simulink model "ev_tms_v4_2022"  (R2023a)
settings: Solver=VariableStepAuto  StartTime=0.0  StopTime=inf  RelTol=1e-3  AbsTol=1e-3
model workspace: external: MATLAB File /Users/rossschrader/Documents/GitHub/RL_EV_TMS/blower_control/power_comparison/ev_tms_v4_params.m (data not in the file)
undefined symbols (not defined in the file): ac_onoff, battery_C1_LUT, battery_capacity_LUT, battery_cell_cp, battery_cell_mass, battery_Em_LUT, battery_N_cells, battery_Qe_init, battery_R0_LUT, battery_R1_LUT, battery_SOC_LUT, battery_T_init, battery_temperature_LUT, bulb, cabin_duct_area, cabin_T_init, chiller_area_primary, chiller_N_baffles, chiller_N_tubes, chiller_tube_D, chiller_tube_L, chiller_wall_conductivity, chiller_wall_thickness, compressor_rpm_LUT, condenser_air_area_flow, condenser_air_area_primary, condenser_W, condenser_wall_conductivity, condenser_wall_thickness, coolant_channel_D, coolant_pipe_D, coolant_T_init, coolant_tank_area, coolant_tank_volume, coolant_valve_D_ratio_max, coolant_valve_D_ratio_min, coolant_valve_displacement, coolant_valve_S_max, evaporator_air_area_flow, evaporator_air_area_primary, evaporator_P_target, evaporator_W, evaporator_wall_conductivity, evaporator_wall_thickness, outlet, pump_speed_max, radiator_air_area_flow, radiator_air_area_primary, radiator_W, radiator_wall_conductivity, radiator_wall_thickness, refrigerant_alpha_init, refrigerant_pipe_D, T_env, T_setpoint
libraries: fl_lib x221, nesl_utility x79, SimscapeFluids_lib x25, LiBatteryElements_lib x16, sdl_lib x3, slpidlib x2, simulink x1, rllib x1, autolibshared x1, SignalEditorBlockLib x1
(part 7 of 7)

== system ev_tms_v4_2022/Environment/Parallel-Serial Mode Valve/Battery Coolant Tank Heat Transfer ==
  Convective Heat Transfer : fl_lib/Thermal/Thermal Elements/Convective Heat Transfer  thermal_type=foundation.enum.constant_variable.constant  area=3 * coolant_tank_area m^2  heat_tr_coeff=20 W/(m^2 * K)  min_heat_tr_coeff=1e-3 W/(K*m^2)  T_specify=off  T_priority=None  T=0 K  T_nominal_specify=off  T_nominal_unit=K  T_nominal_value=1  Q_specify=off  Q_priority=None  Q=0 W  Q_nominal_specify=off  Q_nominal_unit=W  Q_nominal_value=1
  Convective Heat Transfer1 : fl_lib/Thermal/Thermal Elements/Convective Heat Transfer  thermal_type=foundation.enum.constant_variable.constant  area=3 * coolant_tank_area m^2  heat_tr_coeff=20 W/(m^2 * K)  min_heat_tr_coeff=1e-3 W/(K*m^2)  T_specify=off  T_priority=None  T=0 K  T_nominal_specify=off  T_nominal_unit=K  T_nominal_value=1  Q_specify=off  Q_priority=None  Q=0 W  Q_nominal_specify=off  Q_nominal_unit=W  Q_nominal_value=1
  Environment Temperature : fl_lib/Thermal/Thermal Sources/Controlled Temperature Source
  Simulink-PS Converter : nesl_utility/Simulink-PS Converter  PhysicalDomain=network_engine_domain  SubClassName=ps_input  LeftPortType=input  RightPortType=output  PseudoPeriodic=off  Frequencies=[]  NoiseDistribution=none  NoiseParameters=[]  Unit=degC  AffineConversion=on  FilteringAndDerivatives=provide  SimscapeFilterOrder=1  InputFilterTimeConstant=0.001  UdotUserProvided=0
  Thermal Reference : fl_lib/Thermal/Thermal Elements/Thermal Reference
  A : PMIOPort  Side=Left
  B : PMIOPort  Port=2  Side=Left
  wires:
  [T_env] -> Simulink-PS Converter/1
  connections:
  Environment Temperature/LConn1 -- Convective Heat Transfer/RConn1 -- Convective Heat Transfer1/RConn1
  Thermal Reference/LConn1 -- Environment Temperature/RConn2
  Simulink-PS Converter/RConn1 -- Environment Temperature/RConn1
  B/RConn1 -- Convective Heat Transfer1/LConn1
  Convective Heat Transfer/LConn1 -- A/RConn1

== system ev_tms_v4_2022/Environment/Parallel-Serial Mode Valve/Motor Coolant Tank Heat Transfer ==
  Convective Heat Transfer : fl_lib/Thermal/Thermal Elements/Convective Heat Transfer  thermal_type=foundation.enum.constant_variable.constant  area=3 * coolant_tank_area m^2  heat_tr_coeff=20 W/(m^2 * K)  min_heat_tr_coeff=1e-3 W/(K*m^2)  T_specify=off  T_priority=None  T=0 K  T_nominal_specify=off  T_nominal_unit=K  T_nominal_value=1  Q_specify=off  Q_priority=None  Q=0 W  Q_nominal_specify=off  Q_nominal_unit=W  Q_nominal_value=1
  Convective Heat Transfer1 : fl_lib/Thermal/Thermal Elements/Convective Heat Transfer  thermal_type=foundation.enum.constant_variable.constant  area=3 * coolant_tank_area m^2  heat_tr_coeff=20 W/(m^2 * K)  min_heat_tr_coeff=1e-3 W/(K*m^2)  T_specify=off  T_priority=None  T=0 K  T_nominal_specify=off  T_nominal_unit=K  T_nominal_value=1  Q_specify=off  Q_priority=None  Q=0 W  Q_nominal_specify=off  Q_nominal_unit=W  Q_nominal_value=1
  Environment Temperature : fl_lib/Thermal/Thermal Sources/Controlled Temperature Source
  Simulink-PS Converter : nesl_utility/Simulink-PS Converter  PhysicalDomain=network_engine_domain  SubClassName=ps_input  LeftPortType=input  RightPortType=output  PseudoPeriodic=off  Frequencies=[]  NoiseDistribution=none  NoiseParameters=[]  Unit=degC  AffineConversion=on  FilteringAndDerivatives=provide  SimscapeFilterOrder=1  InputFilterTimeConstant=0.001  UdotUserProvided=0
  Thermal Reference : fl_lib/Thermal/Thermal Elements/Thermal Reference
  A : PMIOPort  Side=Right
  B : PMIOPort  Port=2  Side=Right
  wires:
  [T_env] -> Simulink-PS Converter/1
  connections:
  Simulink-PS Converter/RConn1 -- Environment Temperature/RConn1
  Thermal Reference/LConn1 -- Environment Temperature/RConn2
  Convective Heat Transfer/RConn1 -- Environment Temperature/LConn1 -- Convective Heat Transfer1/RConn1
  B/RConn1 -- Convective Heat Transfer1/LConn1
  A/RConn1 -- Convective Heat Transfer/LConn1

== system ev_tms_v4_2022/Environment/Radiator/Ram Pressure ==
  1/2 : fl_lib/Physical Signals/Functions/PS Gain  gain=0.5
  Controlled Pressure Source (MA) : fl_lib/Moist Air/Sources/Controlled Pressure Source (MA)  power_spec=foundation.enum.power_spec.isentropic  area_A=cabin_duct_area m^2  area_B=cabin_duct_area m^2
      settings: InternalSimscapePortConfiguration="{\"Bottom\":[],\"Left\":[{\"id\":\"A\",\"label\":\"A\",\"type\":\"foundation.moist_air.moist_air\"},{\"id\":\"P\",\"label\":\"P\",\"type\":\"input\"}],\"Right\":[{\"id\":\"B\",\"label\":\"B\",\"type\":\"foundation.moist_air.moist_air\"}],\"Top\":[]}"
  PS Product : fl_lib/Physical Signals/Functions/PS Product
  Thermodynamic Properties Sensor (MA) : fl_lib/Moist Air/Sensors/Thermodynamic Properties Sensor (MA)  measurement_mass_spec=foundation.enum.measurement_mass_spec.mixture  enthalpy=true  density=true  specific_heat=true  entropy=true
      settings: InternalSimscapePortConfiguration="{\"Bottom\":[{\"id\":\"CP\",\"label\":\"cp\",\"type\":\"output\"},{\"id\":\"S\",\"label\":\"s\",\"type\":\"output\"}],\"Left\":[{\"id\":\"A\",\"label\":\"A\",\"type\":\"foundation.moist_air.moist_air\"}],\"Right\":[{\"id\":\"H\",\"label\":\"h\",\"type\":\"output\"},{\"id\":\"RHO\",\"label\":\"ρ\",\"type\":\"output\"}],\"Top\":[]}"
  sqr : fl_lib/Physical Signals/Functions/PS Math Function  fcn_choice=foundation.enum.math_function.square  v=1
  A : PMIOPort  Side=Left
  V : PMIOPort  Port=2  Side=Left
  B : PMIOPort  Port=3  Side=Right
  connections:
  Controlled Pressure Source (MA)/RConn1 -- B/RConn1
  Controlled Pressure Source (MA)/LConn1 -- A/RConn1 -- Thermodynamic Properties Sensor (MA)/LConn1
  PS Product/RConn1 -- Controlled Pressure Source (MA)/LConn2
  1/2/RConn1 -- PS Product/LConn1
  sqr/RConn1 -- 1/2/LConn1
  V/RConn1 -- sqr/LConn1
  Thermodynamic Properties Sensor (MA)/RConn2 -- PS Product/LConn2

== system ev_tms_v4_2022/Environment/Radiator/SC1 ==
  Absolute Reference (TL) : fl_lib/Thermal Liquid/Elements/Absolute Reference (TL)
  Mass & Energy Flow Rate Sensor (TL) : fl_lib/Thermal Liquid/Sensors/Flow Rate Sensor (TL)  mass_flow_measure=true  volumetric_flow_measure=false  energy_flow_measure=true
      settings: InternalSimscapePortConfiguration="{\"Bottom\":[{\"id\":\"PHI\",\"label\":\"φ\",\"type\":\"output\"}],\"Left\":[{\"id\":\"A\",\"label\":\"A\",\"type\":\"foundation.thermal_liquid.thermal_liquid\"}],\"Right\":[{\"id\":\"B\",\"label\":\"B\",\"type\":\"foundation.thermal_liquid.thermal_liquid\"},{\"id\":\"M\",\"label\":\"M\",\"type\":\"output\"}],\"Top\":[]}"
  PS-Simulink Converter : nesl_utility/PS-Simulink Converter  PhysicalDomain=network_engine_domain  SubClassName=ps_output  LeftPortType=input  RightPortType=output  PseudoPeriodic=off  Frequencies=[]  VectorFormat=1-D array  Unit=W  AffineConversion=off
  Pressure & Temperature Sensor (TL) : fl_lib/Thermal Liquid/Sensors/Pressure & Temperature Sensor (TL)  reference=foundation.enum.MeasurementReference.difference  pressure=true  pressure_spec=foundation.enum.PressureMeasementSpec.Absolute  temperature=true
      settings: InternalSimscapePortConfiguration="{\"Bottom\":[{\"id\":\"T\",\"label\":\"T\",\"type\":\"output\"}],\"Left\":[{\"id\":\"A\",\"label\":\"A\",\"type\":\"foundation.thermal_liquid.thermal_liquid\"}],\"Right\":[{\"id\":\"B\",\"label\":\"B\",\"type\":\"foundation.thermal_liquid.thermal_liquid\"},{\"id\":\"P\",\"label\":\"P\",\"type\":\"output\"}],\"Top\":[]}"
  B : PMIOPort  Side=Left
  A : PMIOPort  Port=2  Side=Right
  tag scope: Phi_rad_in=global
  wires:
  PS-Simulink Converter/1 -> [Phi_rad_in]
  connections:
  Pressure & Temperature Sensor (TL)/LConn1 -- A/RConn1 -- Mass & Energy Flow Rate Sensor (TL)/LConn1
  Mass & Energy Flow Rate Sensor (TL)/RConn1 -- B/RConn1
  Absolute Reference (TL)/LConn1 -- Pressure & Temperature Sensor (TL)/RConn1
  Mass & Energy Flow Rate Sensor (TL)/RConn3 -- PS-Simulink Converter/LConn1

== system ev_tms_v4_2022/Environment/Radiator/SC2 ==
  Absolute Reference (TL) : fl_lib/Thermal Liquid/Elements/Absolute Reference (TL)
  Mass & Energy Flow Rate Sensor (TL) : fl_lib/Thermal Liquid/Sensors/Flow Rate Sensor (TL)  mass_flow_measure=true  volumetric_flow_measure=false  energy_flow_measure=true
      settings: InternalSimscapePortConfiguration="{\"Bottom\":[{\"id\":\"PHI\",\"label\":\"φ\",\"type\":\"output\"}],\"Left\":[{\"id\":\"A\",\"label\":\"A\",\"type\":\"foundation.thermal_liquid.thermal_liquid\"}],\"Right\":[{\"id\":\"B\",\"label\":\"B\",\"type\":\"foundation.thermal_liquid.thermal_liquid\"},{\"id\":\"M\",\"label\":\"M\",\"type\":\"output\"}],\"Top\":[]}"
  PS-Simulink Converter : nesl_utility/PS-Simulink Converter  PhysicalDomain=network_engine_domain  SubClassName=ps_output  LeftPortType=input  RightPortType=output  PseudoPeriodic=off  Frequencies=[]  VectorFormat=1-D array  Unit=W  AffineConversion=off
  Pressure & Temperature Sensor (TL) : fl_lib/Thermal Liquid/Sensors/Pressure & Temperature Sensor (TL)  reference=foundation.enum.MeasurementReference.difference  pressure=true  pressure_spec=foundation.enum.PressureMeasementSpec.Absolute  temperature=true
      settings: InternalSimscapePortConfiguration="{\"Bottom\":[{\"id\":\"T\",\"label\":\"T\",\"type\":\"output\"}],\"Left\":[{\"id\":\"A\",\"label\":\"A\",\"type\":\"foundation.thermal_liquid.thermal_liquid\"}],\"Right\":[{\"id\":\"B\",\"label\":\"B\",\"type\":\"foundation.thermal_liquid.thermal_liquid\"},{\"id\":\"P\",\"label\":\"P\",\"type\":\"output\"}],\"Top\":[]}"
  B : PMIOPort  Side=Left
  A : PMIOPort  Port=2  Side=Right
  tag scope: Phi_rad_out=global
  wires:
  PS-Simulink Converter/1 -> [Phi_rad_out]
  connections:
  Pressure & Temperature Sensor (TL)/LConn1 -- A/RConn1 -- Mass & Energy Flow Rate Sensor (TL)/LConn1
  Mass & Energy Flow Rate Sensor (TL)/RConn1 -- B/RConn1
  Absolute Reference (TL)/LConn1 -- Pressure & Temperature Sensor (TL)/RConn1
  Mass & Energy Flow Rate Sensor (TL)/RConn3 -- PS-Simulink Converter/LConn1

== system ev_tms_v4_2022/Reward/Temp Reward/If Action Subsystem11 ==
  Action Port : ActionPort  ActionPortLabel=else
  Constant : Constant  Value=15
  Out1 : Outport
  wires:
  Constant/1 -> Out1/1

== system ev_tms_v4_2022/Reward/Temp Reward/If Action Subsystem9 ==
  Input : Inport
  Action Port : ActionPort  ActionPortLabel=if(u1 > 0.5)
  Add : Sum
  Constant : Constant  Value=-10
  Gain : Gain  Gain=-10
  Out1 : Outport
  wires:
  Input/1 -> Gain/1
  Gain/1 -> Add/1
  Constant/1 -> Add/2
  Add/1 -> Out1/1

== system ev_tms_v4_2022/Scenario/Power Demand/Derivative ==
  V : Inport
  Gain : Gain  Gain=tau
  Integrator : Integrator
  Sum : Sum  Inputs=|+-
  A : Outport
  wires:
  V/1 -> Sum/1
  Sum/1 -> Gain/1
  Gain/1 -> Integrator/1, A/1
  Integrator/1 -> Sum/2

== system ev_tms_v4_2022/Controls/Fan Control/Condenser Requirement/Relay Level 1 ==
  in : Inport
  high : Inport  Port=2
  low : Inport  Port=3
  Data Type Conversion : DataTypeConversion  SaturateOnIntegerOverflow=off  RndMeth=Floor
  Relational Operator : RelationalOperator  OutDataTypeStr=boolean  RndMeth=Simplest  InputSameDT=off
  Relational Operator1 : RelationalOperator  Operator=>  OutDataTypeStr=boolean  RndMeth=Simplest  InputSameDT=off
  Relay : Relay  OnSwitchValue=1.5  OffSwitchValue=0.5
  Sum : Sum  Inputs=|++
  out : Outport
  wires:
  Sum/1 -> Data Type Conversion/1
  Data Type Conversion/1 -> Relay/1
  Relational Operator1/1 -> Sum/2
  Relational Operator/1 -> Sum/1
  Relay/1 -> out/1
  low/1 -> Relational Operator1/2
  high/1 -> Relational Operator/2
  in/1 -> Relational Operator/1, Relational Operator1/1

== system ev_tms_v4_2022/Controls/Fan Control/Condenser Requirement/Relay Level 2 ==
  in : Inport
  high : Inport  Port=2
  low : Inport  Port=3
  Data Type Conversion : DataTypeConversion  SaturateOnIntegerOverflow=off  RndMeth=Floor
  Relational Operator : RelationalOperator  OutDataTypeStr=boolean  RndMeth=Simplest  InputSameDT=off
  Relational Operator1 : RelationalOperator  Operator=>  OutDataTypeStr=boolean  RndMeth=Simplest  InputSameDT=off
  Relay : Relay  OnSwitchValue=1.5  OffSwitchValue=0.5
  Sum : Sum  Inputs=|++
  out : Outport
  wires:
  Sum/1 -> Data Type Conversion/1
  Data Type Conversion/1 -> Relay/1
  Relational Operator1/1 -> Sum/2
  Relational Operator/1 -> Sum/1
  Relay/1 -> out/1
  low/1 -> Relational Operator1/2
  high/1 -> Relational Operator/2
  in/1 -> Relational Operator/1, Relational Operator1/1

== system ev_tms_v4_2022/Controls/Fan Control/Condenser Requirement/Relay Level 3 ==
  in : Inport
  high : Inport  Port=2
  low : Inport  Port=3
  Data Type Conversion : DataTypeConversion  SaturateOnIntegerOverflow=off  RndMeth=Floor
  Relational Operator : RelationalOperator  OutDataTypeStr=boolean  RndMeth=Simplest  InputSameDT=off
  Relational Operator1 : RelationalOperator  Operator=>  OutDataTypeStr=boolean  RndMeth=Simplest  InputSameDT=off
  Relay : Relay  OnSwitchValue=1.5  OffSwitchValue=0.5
  Sum : Sum  Inputs=|++
  out : Outport
  wires:
  Sum/1 -> Data Type Conversion/1
  Data Type Conversion/1 -> Relay/1
  Relational Operator1/1 -> Sum/2
  Relational Operator/1 -> Sum/1
  Relay/1 -> out/1
  low/1 -> Relational Operator1/2
  high/1 -> Relational Operator/2
  in/1 -> Relational Operator/1, Relational Operator1/1

== system ev_tms_v4_2022/Environment/Battery/Pack 1/Lithium Cell 1RC ==
  note: Power
      | Losses
  C1 : LiBatteryElements_lib/C_table  C_Table=C1_LUT F  SOC_Table=SOC_LUT  Temp_Table=Temperature_LUT K  v0=0 V
      settings: InternalSimscapePortConfiguration="{\"Bottom\":[],\"Left\":[{\"id\":\"p\",\"label\":\"+\",\"type\":\"foundation.electrical.electrical\"},{\"id\":\"T\",\"label\":\"T\",\"type\":\"input\"},{\"id\":\"SOC\",\"label\":\"SOC\",\"type\":\"input\"}],\"Right\":[{\"id\":\"n\",\"label\":\"-\",\"type\":\"foundation.electrical.electrical\"}],\"Top\":[]}"
  Em_table : LiBatteryElements_lib/Em_table  C_Table=Capacity_LUT hr*A  Em_Table=Em_LUT V  SOC_Table=SOC_LUT  Temp_Table=Temperature_LUT K  Qinit=Qe_init hr*A
      settings: InternalSimscapePortConfiguration="{\"Bottom\":[],\"Left\":[{\"id\":\"p\",\"label\":\"+\",\"type\":\"foundation.electrical.electrical\"},{\"id\":\"C\",\"label\":\"C\",\"type\":\"output\"},{\"id\":\"SOC\",\"label\":\"SOC\",\"type\":\"output\"}],\"Right\":[{\"id\":\"n\",\"label\":\"-\",\"type\":\"foundation.electrical.electrical\"},{\"id\":\"T\",\"label\":\"T\",\"type\":\"input\"}],\"Top\":[]}"
  Power Sum : fl_lib/Physical Signals/Functions/PS Add
  R0 : LiBatteryElements_lib/R_table  R_Table=R0_LUT Ohm  SOC_Table=SOC_LUT  Temp_Table=Temperature_LUT K
      settings: InternalSimscapePortConfiguration="{\"Bottom\":[],\"Left\":[{\"id\":\"p\",\"label\":\"+\",\"type\":\"foundation.electrical.electrical\"},{\"id\":\"T\",\"label\":\"T\",\"type\":\"input\"},{\"id\":\"SOC\",\"label\":\"SOC\",\"type\":\"input\"}],\"Right\":[{\"id\":\"n\",\"label\":\"-\",\"type\":\"foundation.electrical.electrical\"},{\"id\":\"pow\",\"label\":\"POW\",\"type\":\"output\"}],\"Top\":[]}"
  R1 : LiBatteryElements_lib/R_table  R_Table=R1_LUT Ohm  SOC_Table=SOC_LUT  Temp_Table=Temperature_LUT K
      settings: InternalSimscapePortConfiguration="{\"Bottom\":[],\"Left\":[{\"id\":\"p\",\"label\":\"+\",\"type\":\"foundation.electrical.electrical\"},{\"id\":\"T\",\"label\":\"T\",\"type\":\"input\"},{\"id\":\"SOC\",\"label\":\"SOC\",\"type\":\"input\"}],\"Right\":[{\"id\":\"n\",\"label\":\"-\",\"type\":\"foundation.electrical.electrical\"},{\"id\":\"pow\",\"label\":\"POW\",\"type\":\"output\"}],\"Top\":[]}"
  P : PMIOPort  Side=Left
  + : PMIOPort  Port=2  Side=Left
  T : PMIOPort  Port=3  Side=Right
  - : PMIOPort  Port=4  Side=Right
  connections:
  R1/RConn2 -- Power Sum/LConn1
  Power Sum/LConn2 -- R0/RConn2
  P/RConn1 -- Power Sum/RConn1
  +/RConn1 -- R0/RConn1
  T/RConn1 -- Em_table/RConn2 -- R0/LConn2 -- C1/LConn2 -- R1/LConn2
  Em_table/LConn1 -- C1/LConn1 -- R1/LConn1
  C1/RConn1 -- R1/RConn1 -- R0/LConn1
  Em_table/RConn1 -- -/RConn1
  C1/LConn3 -- Em_table/LConn3 -- R1/LConn3 -- R0/LConn3

== system ev_tms_v4_2022/Environment/Battery/Pack 1/Thermal Model ==
  Battery Thermal Mass : fl_lib/Thermal/Thermal Elements/Thermal Mass  mass_type=foundation.enum.constant_variable.constant  mass=cell_mass*Ncells kg  sp_heat=cell_Cp_heat J/kg/K  mass_min=1e-6 kg  num_ports=foundation.enum.numPorts2.one  m_specify=off  m_priority=High  m=1 kg  m_nominal_specify=off  m_nominal_unit=kg  m_nominal_value=1  T_specify=on  T_priority=High  T=T_init K  T_nominal_specify=off  T_nominal_unit=K  T_nominal_value=1  Q_specify=off  Q_priority=None  Q=0 W  Q_nominal_specify=off  Q_nominal_unit=W  Q_nominal_value=1
  Controlled Heat Flow Rate Source : fl_lib/Thermal/Thermal Sources/Controlled Heat Flow Rate Source
  Temperature Sensor : fl_lib/Thermal/Thermal Sensors/Temperature Sensor  temperature_measure=foundation.enum.MeasurementReference.difference
  Thermal Reference : fl_lib/Thermal/Thermal Elements/Thermal Reference
  Thermal Reference2 : fl_lib/Thermal/Thermal Elements/Thermal Reference
  H : PMIOPort  Side=Left
  Pxn : PMIOPort  Port=2  Side=Left
  T : PMIOPort  Port=3  Side=Right
  connections:
  H/RConn1 -- Controlled Heat Flow Rate Source/LConn1 -- Battery Thermal Mass/LConn1 -- Temperature Sensor/LConn1
  Pxn/RConn1 -- Controlled Heat Flow Rate Source/RConn1
  Controlled Heat Flow Rate Source/RConn2 -- Thermal Reference2/LConn1
  Thermal Reference/LConn1 -- Temperature Sensor/RConn1
  T/RConn1 -- Temperature Sensor/RConn2

== system ev_tms_v4_2022/Environment/Battery/Pack 2/Lithium Cell 1RC ==
  note: Power
      | Losses
  C1 : LiBatteryElements_lib/C_table  C_Table=C1_LUT F  SOC_Table=SOC_LUT  Temp_Table=Temperature_LUT K  v0=0 V
      settings: InternalSimscapePortConfiguration="{\"Bottom\":[],\"Left\":[{\"id\":\"p\",\"label\":\"+\",\"type\":\"foundation.electrical.electrical\"},{\"id\":\"T\",\"label\":\"T\",\"type\":\"input\"},{\"id\":\"SOC\",\"label\":\"SOC\",\"type\":\"input\"}],\"Right\":[{\"id\":\"n\",\"label\":\"-\",\"type\":\"foundation.electrical.electrical\"}],\"Top\":[]}"
  Em_table : LiBatteryElements_lib/Em_table  C_Table=Capacity_LUT hr*A  Em_Table=Em_LUT V  SOC_Table=SOC_LUT  Temp_Table=Temperature_LUT K  Qinit=Qe_init hr*A
      settings: InternalSimscapePortConfiguration="{\"Bottom\":[],\"Left\":[{\"id\":\"p\",\"label\":\"+\",\"type\":\"foundation.electrical.electrical\"},{\"id\":\"C\",\"label\":\"C\",\"type\":\"output\"},{\"id\":\"SOC\",\"label\":\"SOC\",\"type\":\"output\"}],\"Right\":[{\"id\":\"n\",\"label\":\"-\",\"type\":\"foundation.electrical.electrical\"},{\"id\":\"T\",\"label\":\"T\",\"type\":\"input\"}],\"Top\":[]}"
  Power Sum : fl_lib/Physical Signals/Functions/PS Add
  R0 : LiBatteryElements_lib/R_table  R_Table=R0_LUT Ohm  SOC_Table=SOC_LUT  Temp_Table=Temperature_LUT K
      settings: InternalSimscapePortConfiguration="{\"Bottom\":[],\"Left\":[{\"id\":\"p\",\"label\":\"+\",\"type\":\"foundation.electrical.electrical\"},{\"id\":\"T\",\"label\":\"T\",\"type\":\"input\"},{\"id\":\"SOC\",\"label\":\"SOC\",\"type\":\"input\"}],\"Right\":[{\"id\":\"n\",\"label\":\"-\",\"type\":\"foundation.electrical.electrical\"},{\"id\":\"pow\",\"label\":\"POW\",\"type\":\"output\"}],\"Top\":[]}"
  R1 : LiBatteryElements_lib/R_table  R_Table=R1_LUT Ohm  SOC_Table=SOC_LUT  Temp_Table=Temperature_LUT K
      settings: InternalSimscapePortConfiguration="{\"Bottom\":[],\"Left\":[{\"id\":\"p\",\"label\":\"+\",\"type\":\"foundation.electrical.electrical\"},{\"id\":\"T\",\"label\":\"T\",\"type\":\"input\"},{\"id\":\"SOC\",\"label\":\"SOC\",\"type\":\"input\"}],\"Right\":[{\"id\":\"n\",\"label\":\"-\",\"type\":\"foundation.electrical.electrical\"},{\"id\":\"pow\",\"label\":\"POW\",\"type\":\"output\"}],\"Top\":[]}"
  P : PMIOPort  Side=Left
  + : PMIOPort  Port=2  Side=Left
  T : PMIOPort  Port=3  Side=Right
  - : PMIOPort  Port=4  Side=Right
  connections:
  R1/RConn2 -- Power Sum/LConn1
  Power Sum/LConn2 -- R0/RConn2
  P/RConn1 -- Power Sum/RConn1
  +/RConn1 -- R0/RConn1
  T/RConn1 -- Em_table/RConn2 -- R0/LConn2 -- C1/LConn2 -- R1/LConn2
  Em_table/LConn1 -- C1/LConn1 -- R1/LConn1
  C1/RConn1 -- R1/RConn1 -- R0/LConn1
  Em_table/RConn1 -- -/RConn1
  C1/LConn3 -- Em_table/LConn3 -- R1/LConn3 -- R0/LConn3

== system ev_tms_v4_2022/Environment/Battery/Pack 2/Thermal Model ==
  Battery Thermal Mass : fl_lib/Thermal/Thermal Elements/Thermal Mass  mass_type=foundation.enum.constant_variable.constant  mass=cell_mass*Ncells kg  sp_heat=cell_Cp_heat J/kg/K  mass_min=1e-6 kg  num_ports=foundation.enum.numPorts2.one  m_specify=off  m_priority=High  m=1 kg  m_nominal_specify=off  m_nominal_unit=kg  m_nominal_value=1  T_specify=on  T_priority=High  T=T_init K  T_nominal_specify=off  T_nominal_unit=K  T_nominal_value=1  Q_specify=off  Q_priority=None  Q=0 W  Q_nominal_specify=off  Q_nominal_unit=W  Q_nominal_value=1
  Controlled Heat Flow Rate Source : fl_lib/Thermal/Thermal Sources/Controlled Heat Flow Rate Source
  Temperature Sensor : fl_lib/Thermal/Thermal Sensors/Temperature Sensor  temperature_measure=foundation.enum.MeasurementReference.difference
  Thermal Reference : fl_lib/Thermal/Thermal Elements/Thermal Reference
  Thermal Reference2 : fl_lib/Thermal/Thermal Elements/Thermal Reference
  H : PMIOPort  Side=Left
  Pxn : PMIOPort  Port=2  Side=Left
  T : PMIOPort  Port=3  Side=Right
  connections:
  H/RConn1 -- Controlled Heat Flow Rate Source/LConn1 -- Battery Thermal Mass/LConn1 -- Temperature Sensor/LConn1
  Pxn/RConn1 -- Controlled Heat Flow Rate Source/RConn1
  Controlled Heat Flow Rate Source/RConn2 -- Thermal Reference2/LConn1
  Thermal Reference/LConn1 -- Temperature Sensor/RConn1
  T/RConn1 -- Temperature Sensor/RConn2

== system ev_tms_v4_2022/Environment/Battery/Pack 3/Lithium Cell 1RC ==
  note: Power
      | Losses
  C1 : LiBatteryElements_lib/C_table  C_Table=C1_LUT F  SOC_Table=SOC_LUT  Temp_Table=Temperature_LUT K  v0=0 V
      settings: InternalSimscapePortConfiguration="{\"Bottom\":[],\"Left\":[{\"id\":\"p\",\"label\":\"+\",\"type\":\"foundation.electrical.electrical\"},{\"id\":\"T\",\"label\":\"T\",\"type\":\"input\"},{\"id\":\"SOC\",\"label\":\"SOC\",\"type\":\"input\"}],\"Right\":[{\"id\":\"n\",\"label\":\"-\",\"type\":\"foundation.electrical.electrical\"}],\"Top\":[]}"
  Em_table : LiBatteryElements_lib/Em_table  C_Table=Capacity_LUT hr*A  Em_Table=Em_LUT V  SOC_Table=SOC_LUT  Temp_Table=Temperature_LUT K  Qinit=Qe_init hr*A
      settings: InternalSimscapePortConfiguration="{\"Bottom\":[],\"Left\":[{\"id\":\"p\",\"label\":\"+\",\"type\":\"foundation.electrical.electrical\"},{\"id\":\"C\",\"label\":\"C\",\"type\":\"output\"},{\"id\":\"SOC\",\"label\":\"SOC\",\"type\":\"output\"}],\"Right\":[{\"id\":\"n\",\"label\":\"-\",\"type\":\"foundation.electrical.electrical\"},{\"id\":\"T\",\"label\":\"T\",\"type\":\"input\"}],\"Top\":[]}"
  Power Sum : fl_lib/Physical Signals/Functions/PS Add
  R0 : LiBatteryElements_lib/R_table  R_Table=R0_LUT Ohm  SOC_Table=SOC_LUT  Temp_Table=Temperature_LUT K
      settings: InternalSimscapePortConfiguration="{\"Bottom\":[],\"Left\":[{\"id\":\"p\",\"label\":\"+\",\"type\":\"foundation.electrical.electrical\"},{\"id\":\"T\",\"label\":\"T\",\"type\":\"input\"},{\"id\":\"SOC\",\"label\":\"SOC\",\"type\":\"input\"}],\"Right\":[{\"id\":\"n\",\"label\":\"-\",\"type\":\"foundation.electrical.electrical\"},{\"id\":\"pow\",\"label\":\"POW\",\"type\":\"output\"}],\"Top\":[]}"
  R1 : LiBatteryElements_lib/R_table  R_Table=R1_LUT Ohm  SOC_Table=SOC_LUT  Temp_Table=Temperature_LUT K
      settings: InternalSimscapePortConfiguration="{\"Bottom\":[],\"Left\":[{\"id\":\"p\",\"label\":\"+\",\"type\":\"foundation.electrical.electrical\"},{\"id\":\"T\",\"label\":\"T\",\"type\":\"input\"},{\"id\":\"SOC\",\"label\":\"SOC\",\"type\":\"input\"}],\"Right\":[{\"id\":\"n\",\"label\":\"-\",\"type\":\"foundation.electrical.electrical\"},{\"id\":\"pow\",\"label\":\"POW\",\"type\":\"output\"}],\"Top\":[]}"
  P : PMIOPort  Side=Left
  + : PMIOPort  Port=2  Side=Left
  T : PMIOPort  Port=3  Side=Right
  - : PMIOPort  Port=4  Side=Right
  connections:
  R0/LConn3 -- R1/LConn3 -- Em_table/LConn3 -- C1/LConn3
  Em_table/RConn1 -- -/RConn1
  R0/LConn1 -- R1/RConn1 -- C1/RConn1
  R1/LConn1 -- C1/LConn1 -- Em_table/LConn1
  R1/LConn2 -- C1/LConn2 -- R0/LConn2 -- Em_table/RConn2 -- T/RConn1
  +/RConn1 -- R0/RConn1
  P/RConn1 -- Power Sum/RConn1
  Power Sum/LConn2 -- R0/RConn2
  R1/RConn2 -- Power Sum/LConn1

== system ev_tms_v4_2022/Environment/Battery/Pack 3/Thermal Model ==
  Battery Thermal Mass : fl_lib/Thermal/Thermal Elements/Thermal Mass  mass_type=foundation.enum.constant_variable.constant  mass=cell_mass*Ncells kg  sp_heat=cell_Cp_heat J/kg/K  mass_min=1e-6 kg  num_ports=foundation.enum.numPorts2.one  m_specify=off  m_priority=High  m=1 kg  m_nominal_specify=off  m_nominal_unit=kg  m_nominal_value=1  T_specify=on  T_priority=High  T=T_init K  T_nominal_specify=off  T_nominal_unit=K  T_nominal_value=1  Q_specify=off  Q_priority=None  Q=0 W  Q_nominal_specify=off  Q_nominal_unit=W  Q_nominal_value=1
  Controlled Heat Flow Rate Source : fl_lib/Thermal/Thermal Sources/Controlled Heat Flow Rate Source
  Temperature Sensor : fl_lib/Thermal/Thermal Sensors/Temperature Sensor  temperature_measure=foundation.enum.MeasurementReference.difference
  Thermal Reference : fl_lib/Thermal/Thermal Elements/Thermal Reference
  Thermal Reference2 : fl_lib/Thermal/Thermal Elements/Thermal Reference
  H : PMIOPort  Side=Left
  Pxn : PMIOPort  Port=2  Side=Left
  T : PMIOPort  Port=3  Side=Right
  connections:
  T/RConn1 -- Temperature Sensor/RConn2
  Thermal Reference/LConn1 -- Temperature Sensor/RConn1
  Controlled Heat Flow Rate Source/RConn2 -- Thermal Reference2/LConn1
  Pxn/RConn1 -- Controlled Heat Flow Rate Source/RConn1
  Temperature Sensor/LConn1 -- Battery Thermal Mass/LConn1 -- Controlled Heat Flow Rate Source/LConn1 -- H/RConn1

== system ev_tms_v4_2022/Environment/Battery/Pack 4/Lithium Cell 1RC ==
  note: Power
      | Losses
  C1 : LiBatteryElements_lib/C_table  C_Table=C1_LUT F  SOC_Table=SOC_LUT  Temp_Table=Temperature_LUT K  v0=0 V
      settings: InternalSimscapePortConfiguration="{\"Bottom\":[],\"Left\":[{\"id\":\"p\",\"label\":\"+\",\"type\":\"foundation.electrical.electrical\"},{\"id\":\"T\",\"label\":\"T\",\"type\":\"input\"},{\"id\":\"SOC\",\"label\":\"SOC\",\"type\":\"input\"}],\"Right\":[{\"id\":\"n\",\"label\":\"-\",\"type\":\"foundation.electrical.electrical\"}],\"Top\":[]}"
  Em_table : LiBatteryElements_lib/Em_table  C_Table=Capacity_LUT hr*A  Em_Table=Em_LUT V  SOC_Table=SOC_LUT  Temp_Table=Temperature_LUT K  Qinit=Qe_init hr*A
      settings: InternalSimscapePortConfiguration="{\"Bottom\":[],\"Left\":[{\"id\":\"p\",\"label\":\"+\",\"type\":\"foundation.electrical.electrical\"},{\"id\":\"C\",\"label\":\"C\",\"type\":\"output\"},{\"id\":\"SOC\",\"label\":\"SOC\",\"type\":\"output\"}],\"Right\":[{\"id\":\"n\",\"label\":\"-\",\"type\":\"foundation.electrical.electrical\"},{\"id\":\"T\",\"label\":\"T\",\"type\":\"input\"}],\"Top\":[]}"
  Power Sum : fl_lib/Physical Signals/Functions/PS Add
  R0 : LiBatteryElements_lib/R_table  R_Table=R0_LUT Ohm  SOC_Table=SOC_LUT  Temp_Table=Temperature_LUT K
      settings: InternalSimscapePortConfiguration="{\"Bottom\":[],\"Left\":[{\"id\":\"p\",\"label\":\"+\",\"type\":\"foundation.electrical.electrical\"},{\"id\":\"T\",\"label\":\"T\",\"type\":\"input\"},{\"id\":\"SOC\",\"label\":\"SOC\",\"type\":\"input\"}],\"Right\":[{\"id\":\"n\",\"label\":\"-\",\"type\":\"foundation.electrical.electrical\"},{\"id\":\"pow\",\"label\":\"POW\",\"type\":\"output\"}],\"Top\":[]}"
  R1 : LiBatteryElements_lib/R_table  R_Table=R1_LUT Ohm  SOC_Table=SOC_LUT  Temp_Table=Temperature_LUT K
      settings: InternalSimscapePortConfiguration="{\"Bottom\":[],\"Left\":[{\"id\":\"p\",\"label\":\"+\",\"type\":\"foundation.electrical.electrical\"},{\"id\":\"T\",\"label\":\"T\",\"type\":\"input\"},{\"id\":\"SOC\",\"label\":\"SOC\",\"type\":\"input\"}],\"Right\":[{\"id\":\"n\",\"label\":\"-\",\"type\":\"foundation.electrical.electrical\"},{\"id\":\"pow\",\"label\":\"POW\",\"type\":\"output\"}],\"Top\":[]}"
  P : PMIOPort  Side=Left
  + : PMIOPort  Port=2  Side=Left
  T : PMIOPort  Port=3  Side=Right
  - : PMIOPort  Port=4  Side=Right
  connections:
  R1/RConn2 -- Power Sum/LConn1
  Power Sum/LConn2 -- R0/RConn2
  P/RConn1 -- Power Sum/RConn1
  +/RConn1 -- R0/RConn1
  T/RConn1 -- Em_table/RConn2 -- R0/LConn2 -- C1/LConn2 -- R1/LConn2
  Em_table/LConn1 -- C1/LConn1 -- R1/LConn1
  C1/RConn1 -- R1/RConn1 -- R0/LConn1
  Em_table/RConn1 -- -/RConn1
  C1/LConn3 -- Em_table/LConn3 -- R1/LConn3 -- R0/LConn3

== system ev_tms_v4_2022/Environment/Battery/Pack 4/Thermal Model ==
  Battery Thermal Mass : fl_lib/Thermal/Thermal Elements/Thermal Mass  mass_type=foundation.enum.constant_variable.constant  mass=cell_mass*Ncells kg  sp_heat=cell_Cp_heat J/kg/K  mass_min=1e-6 kg  num_ports=foundation.enum.numPorts2.one  m_specify=off  m_priority=High  m=1 kg  m_nominal_specify=off  m_nominal_unit=kg  m_nominal_value=1  T_specify=on  T_priority=High  T=T_init K  T_nominal_specify=off  T_nominal_unit=K  T_nominal_value=1  Q_specify=off  Q_priority=None  Q=0 W  Q_nominal_specify=off  Q_nominal_unit=W  Q_nominal_value=1
  Controlled Heat Flow Rate Source : fl_lib/Thermal/Thermal Sources/Controlled Heat Flow Rate Source
  Temperature Sensor : fl_lib/Thermal/Thermal Sensors/Temperature Sensor  temperature_measure=foundation.enum.MeasurementReference.difference
  Thermal Reference : fl_lib/Thermal/Thermal Elements/Thermal Reference
  Thermal Reference2 : fl_lib/Thermal/Thermal Elements/Thermal Reference
  H : PMIOPort  Side=Left
  Pxn : PMIOPort  Port=2  Side=Left
  T : PMIOPort  Port=3  Side=Right
  connections:
  H/RConn1 -- Controlled Heat Flow Rate Source/LConn1 -- Battery Thermal Mass/LConn1 -- Temperature Sensor/LConn1
  Pxn/RConn1 -- Controlled Heat Flow Rate Source/RConn1
  Controlled Heat Flow Rate Source/RConn2 -- Thermal Reference2/LConn1
  Thermal Reference/LConn1 -- Temperature Sensor/RConn1
  T/RConn1 -- Temperature Sensor/RConn2
